simulink model "TankPIDCtrl"  (R2023a)
settings: Solver=FixedStepAuto  StartTime=0.0  StopTime=inf  FixedStep=0.1  RelTol=1e-3
model workspace (MAT data in the model file):
  U = 20
libraries: simulink x1, aerolibanimutils x1
settings Model: PacingRate=10  Creator=gener  LastModifiedBy=Magician
settings SolverCC: AutoInsertRateTranBlk=on  InsertRTBMode=Always
settings OptimizationCC: ReuseModelBlockBuffer=off

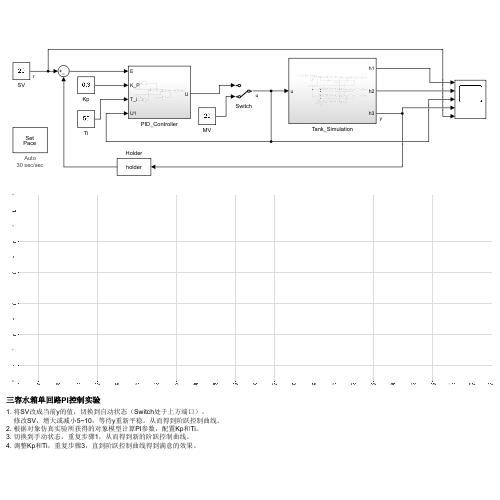
[thumbnail: Simulink's stored preview of the top-level diagram]
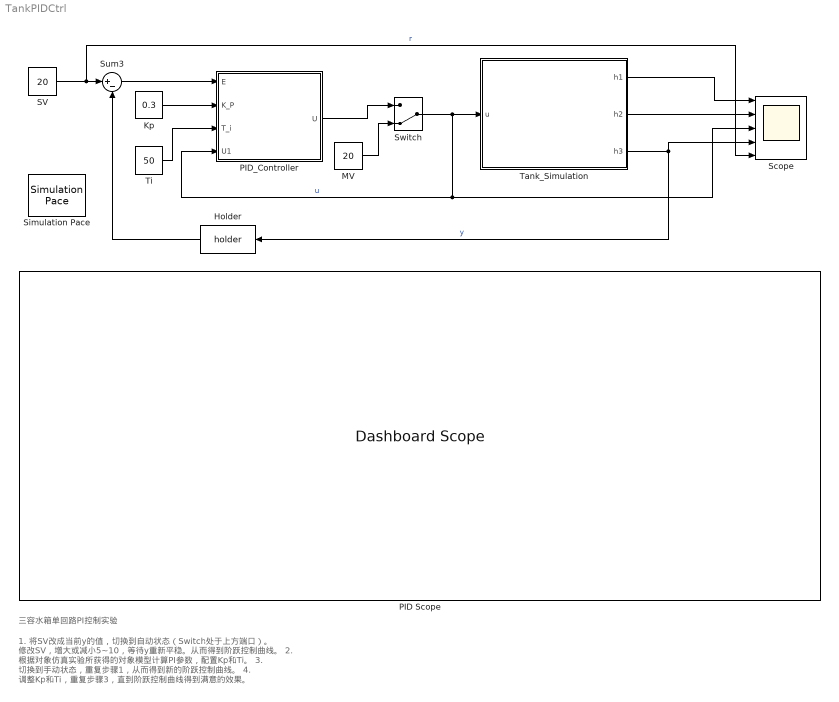
== system TankPIDCtrl ==
  note: 1. 将SV改成当前y的值，切换到自动状态（Switch处于上方端口）。
      | 修改SV，增大或减小5~10，等待y重新平稳。从而得到阶跃控制曲线。
      | 2. 根据对象仿真实验所获得的对象模型计算PI参数，配置Kp和Ti。
      | 3. 切换到手动状态，重复步骤1，从而得到新的阶跃控制曲线。
      | 4. 调整Kp和Ti，重复步骤3，直到阶跃控制曲线得到满意的效果。
  note: 三容水箱单回路PI控制实验
  Holder : S-Function  FunctionName=holder  SFunctionDeploymentMode=off  EnableBusSupport=off
  Kp : Constant  Value=0.3
  MV : Constant  Value=20
  PID Scope : DashboardScope  TimeSpan=1200
  PID_Controller : Subsystem
  SV : Constant  Value=20
  Scope : Scope  NumInputPorts=5
  Simulation Pace : aerolibanimutils/Simulation Pace  SimulationPace=30  SleepMode=Auto  OutputPaceError=off  SampleTime=0.1
  Sum3 : Sum  Inputs=|+-
  Switch : ManualSwitch  CurrentSetting=0
  Tank_Simulation : Subsystem
  Ti : Constant  Value=50
  wires:
  Tank_Simulation/3(h3) -> Scope/4, Holder/1  "y"
  Switch/1 -> Tank_Simulation/1(u), Scope/3, PID_Controller/4(U1)  "u"
  Tank_Simulation/1(h1) -> Scope/1
  Tank_Simulation/2(h2) -> Scope/2
  Sum3/1 -> PID_Controller/1(E)
  Holder/1 -> Sum3/2
  SV/1 -> Scope/5, Sum3/1  "r"
  Kp/1 -> PID_Controller/2(K_P)
  Ti/1 -> PID_Controller/3(T_i)
  PID_Controller/1(U) -> Switch/1
  MV/1 -> Switch/2

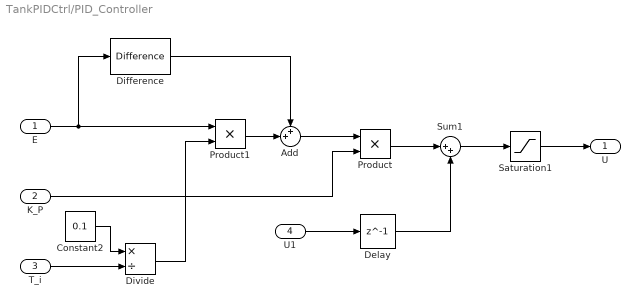
== system TankPIDCtrl/PID_Controller ==
  E : Inport
  K_P : Inport  Port=2
  T_i : Inport  Port=3
  U1 : Inport  Port=4
  Add : Sum  Inputs=++|
  Constant2 : Constant  Value=0.1
  Delay : Delay  DelayLength=1  SampleTime=0.1
  Difference : simulink/Discrete/Difference  ICPrevInput=0.0  OutMin=[]  OutMax=[]  OutDataType=fixdt(1, 16)  OutScaling=2^-10  DoSatur=off
  Divide : Product  Inputs=*/
  Product : Product
  Product1 : Product
  Saturation1 : Saturate  UpperLimit=100  LowerLimit=0
  Sum1 : Sum  Inputs=|++
  U : Outport
  wires:
  E/1 -> Product1/1, Difference/1
  Sum1/1 -> Saturation1/1
  Saturation1/1 -> U/1
  Delay/1 -> Sum1/2
  T_i/1 -> Divide/2
  U1/1 -> Delay/1
  Difference/1 -> Add/1
  Product/1 -> Sum1/1
  Add/1 -> Product/1
  K_P/1 -> Product/2
  Product1/1 -> Add/2
  Divide/1 -> Product1/2
  Constant2/1 -> Divide/1

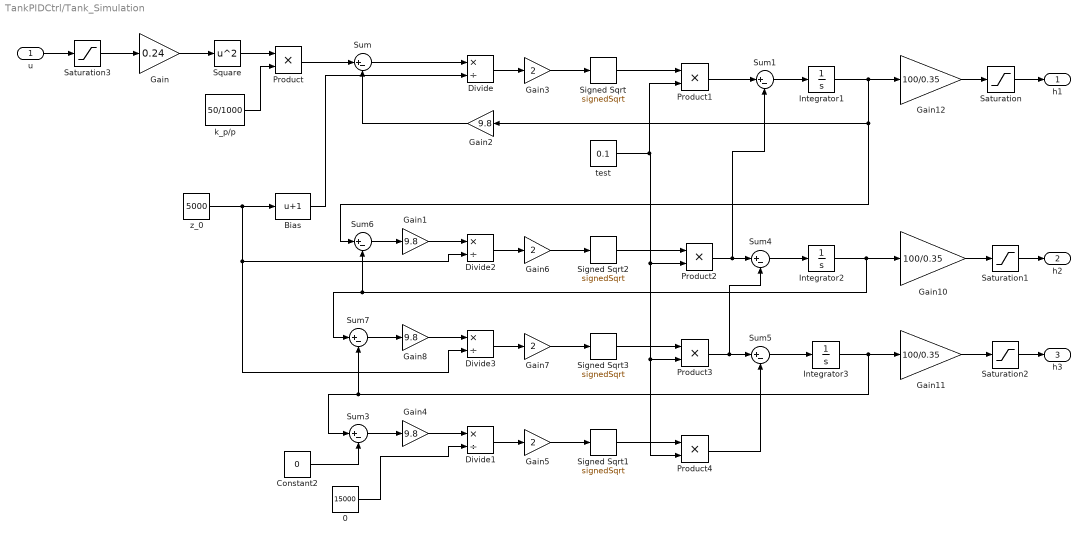
== system TankPIDCtrl/Tank_Simulation ==
  u : Inport
  0 : Constant  Value=15000
  Bias : Bias  Bias=1  SaturateOnIntegerOverflow=off
  Constant2 : Constant  Value=0
  Divide{,1..3} (4 alike) : Product  Inputs=*/
  Gain : Gain  Gain=0.24
  Gain{1..2,4,8} (4 alike) : Gain  Gain=9.8
  Gain10 : Gain  Gain=100/0.35
  Gain11 : Gain  Gain=100/0.35
  Gain12 : Gain  Gain=100/0.35
  Gain{3,5..7} (4 alike) : Gain  Gain=2
  Integrator1 : Integrator
  Integrator2 : Integrator
  Integrator3 : Integrator
  Product{,1..4} (5 alike) : Product
  Saturation{,1..3} (4 alike) : Saturate  UpperLimit=100  LowerLimit=0
  Signed Sqrt{,1..3} (4 alike) : Sqrt  Operator=signedSqrt
  Square : Math  Operator=square
  Sum{,1,3..7} (7 alike) : Sum  Inputs=|+-
  k_p/p : Constant  Value=50/1000
  test : Constant  Value=0.1
  z_0 : Constant  Value=5000
  h1 : Outport
  h2 : Outport  Port=2
  h3 : Outport  Port=3
  wires:
  Signed Sqrt1/1 -> Product4/1
  Integrator1/1 -> Gain12/1, Sum6/1, Gain2/1
  Bias/1 -> Divide/2
  Signed Sqrt2/1 -> Product2/1
  Divide/1 -> Gain3/1
  Sum/1 -> Divide/1
  Sum1/1 -> Integrator1/1
  Product3/1 -> Sum4/2, Sum5/1
  z_0/1 -> Bias/1, Divide3/2, Divide2/2
  Integrator3/1 -> Gain11/1, Sum7/2, Sum3/1
  Gain/1 -> Square/1
  Gain3/1 -> Signed Sqrt/1
  Signed Sqrt/1 -> Product1/1
  Divide1/1 -> Gain5/1
  Constant2/1 -> Sum3/2
  Sum6/1 -> Gain1/1
  Sum4/1 -> Integrator2/1
  Divide2/1 -> Gain6/1
  Integrator2/1 -> Gain10/1, Sum6/2, Sum7/1
  Gain7/1 -> Signed Sqrt3/1
  Signed Sqrt3/1 -> Product3/1
  Sum7/1 -> Gain8/1
  Sum3/1 -> Gain4/1
  Product4/1 -> Sum5/2
  Gain5/1 -> Signed Sqrt1/1
  Product2/1 -> Sum1/2, Sum4/1
  Product1/1 -> Sum1/1
  Sum5/1 -> Integrator3/1
  Gain6/1 -> Signed Sqrt2/1
  Gain4/1 -> Divide1/1
  k_p/p/1 -> Product/2
  Product/1 -> Sum/1
  Square/1 -> Product/1
  Gain8/1 -> Divide3/1
  Divide3/1 -> Gain7/1
  Gain1/1 -> Divide2/1
  Gain2/1 -> Sum/2
  Saturation/1 -> h1/1
  Gain12/1 -> Saturation/1
  Gain10/1 -> Saturation1/1
  Saturation1/1 -> h2/1
  Gain11/1 -> Saturation2/1
  Saturation2/1 -> h3/1
  u/1 -> Saturation3/1
  Saturation3/1 -> Gain/1
  test/1 -> Product3/2, Product4/2, Product2/2, Product1/2
  0/1 -> Divide1/2
